simulink model "LQG_CubeSat"  (R2024a)
settings: Solver=VariableStepAuto  StartTime=0.0  StopTime=100  RelTol=1e-3
values from neighbouring files (symbols this model uses):
  I_rw_zz = 0.02 / 523.59    (= 3.81978265437e-05)    [main_CubeSatControl.m]
  I_s = [I_xx 0 0 ... (first row only)    [main_CubeSatControl.m]
  inv_I_s = inv(I_s)    [main_CubeSatControl.m]
  K_p = [K_p_base*axis_ratio 0 0 ... (first row only)    [main_CubeSatControl.m]
  K_pd = [K_pd_base*axis_ratio 0 0 ... (first row only)    [main_CubeSatControl.m]
  tau_motor_loop = 1    [main_CubeSatControl.m]
libraries: vrlib x1, matrix_library x1, aerolibanimutils x1, simulink x1
settings Model: Creator=joshk  LastModifiedBy=joshk
settings RTWCC: GPUComputeCapability=3.5

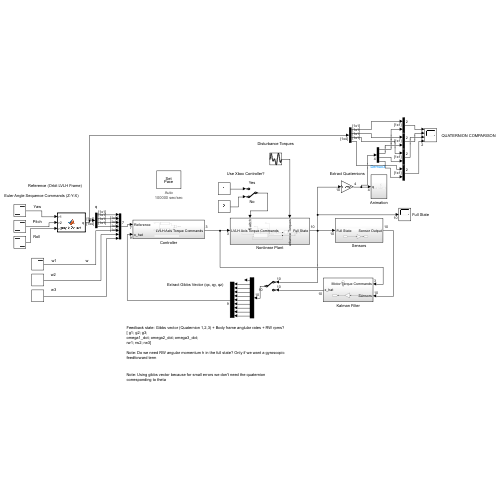
[thumbnail: Simulink's stored preview of the top-level diagram]
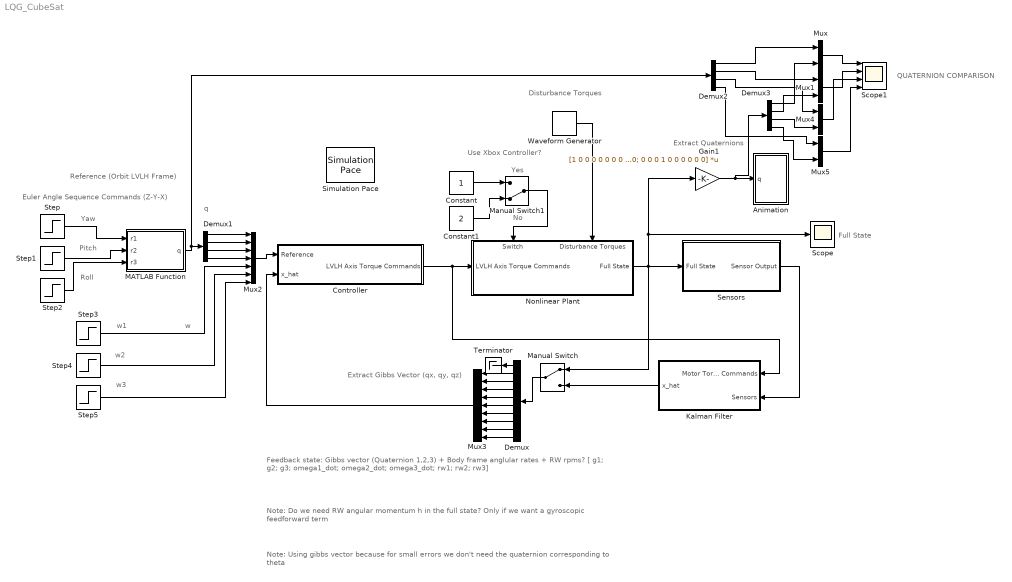
== system LQG_CubeSat ==
  note: QUATERNION COMPARISON
  note: w
  note: q
  note: Disturbance Torques
  note: Note: Using gibbs vector because for small errors we don't need the quaternion corresponding to theta
  note: Full State
  note: Extract Quaternions
  note: Euler Angle Sequence Commands (Z-Y-X)
  note: Note: Do we need RW angular momentum h in the full state? Only if we want a gyroscopic feedforward term
  note: Feedback state: Gibbs vector (Quaternion 1,2,3) + Body frame anglular rates + RW rpms?
      | [ g1; g2; g3;
      | omega1_dot; omega2_dot; omega3_dot;
      | rw1; rw2; rw3]
  note: No
  note: Yes
  note: Use Xbox Controller?
  note: Roll
  note: Pitch
  note: Yaw
  note: Reference (Orbit LVLH Frame)
  note: w2
  note: w3
  note: w1
  note: Extract Gibbs Vector (qx, qy, qz)
  Animation : Subsystem
  Constant : Constant
  Constant1 : Constant  Value=2
  Controller : Subsystem
  Demux : Demux  Outputs=10
  Demux1 : Demux
  Demux2 : Demux
  Demux3 : Demux
  Gain1 : Gain  Gain=[1 0 0 0 0 0 0 0 0 0; 0 1 0 0 0 0 0 0 0 0; 0 0 1 0 0 0 0 0 0 0; 0 0 0 1 0 0 0 0 0 0]  Multiplication=Matrix(K*u) (u vector)
  Kalman Filter : Subsystem
  MATLAB Function : MATLAB Function  TreatAsAtomicUnit=on
  Manual Switch : ManualSwitch
  Manual Switch1 : ManualSwitch  CurrentSetting=0
  Mux{,1,4..5} (4 alike) : Mux  Inputs=2
  Mux2 : Mux  Inputs=7
  Mux3 : Mux  Inputs=9
  Nonlinear Plant : Subsystem
      settings: PortSchema="{\"entries\":[{\"content\":{\"sides\":[{\"content\":{\"connectorIds\":[\"In1\"]},\"type\":\"ConnectorPlacement.EquallySpacedRectSide\",\"uuid\":\"9b91c08c-2a90-4f12-ae99-41b2d0c7dbbf\"},{\"content\":{\"connectorIds\":[\"Out1\"],\"side\":\"RIGHT\"},\"type\":\"ConnectorPlacement.EquallySpacedRectSide\",\"uuid\":\"14ab69da-e910-4abb-8476-8d8dff4f3eb1\"},{\"content\":{\"connectorIds\":[\"In2\",\"In3\"],\"side\":\"TOP\"},\"type\":\"ConnectorPlacement.EquallySpacedRectSide\",\"uuid\":\"c21f965e-6c73-42bc-bf21-433ba90567d6\"}]},\"type\":\"ConnectorPlacement.EquallySpacedConnector\",\"uuid\":\"eb7c3899-db95-4d15-9719-1c6a9ded63d0\"}],\"packageUris\":[\"http://schema.mathworks.com/mf0/Connector/R2020b\"],\"version\":\"1.0\"}"
  Scope : Scope
  Scope1 : Scope  NumInputPorts=4
  Sensors : Subsystem
  Simulation Pace : aerolibanimutils/Simulation Pace  SimulationPace=100000  SleepMode=Auto  OutputPaceError=off  SampleTime=1/50
  Step : Step  Time=2  After=0.1  SampleTime=0
  Step1 : Step  Time=2  After=0.5  SampleTime=0
  Step2 : Step  Time=2  After=-0.3  SampleTime=0
  Step3 : Step  Time=2  After=0  SampleTime=0
  Step4 : Step  Time=2  After=0  SampleTime=0
  Step5 : Step  Time=2  After=0  SampleTime=0
  Terminator : Terminator
  Waveform Generator : simulink/Sources/Waveform Generator  OutMin=[]  OutMax=[]  OutDataTypeStr=double  SelectedSignal=1  BlockNames=MultiportSwitch_e3df3653d217406  SampleTime=0.1
  wires:
  Sensors/1(Sensor Output) -> Kalman Filter/2(Sensors)
  Step1/1 -> MATLAB Function/2(r2)
  Step/1 -> MATLAB Function/1(r1)
  Step2/1 -> MATLAB Function/3(r3)
  Kalman Filter/1(x_hat) -> Manual Switch/2
  Controller/1(LVLH Axis Torque Commands) -> Kalman Filter/1(Motor Torque Commands), Nonlinear Plant/1(LVLH Axis Torque Commands)
  Manual Switch1/1 -> Nonlinear Plant/2(Switch)
  Constant/1 -> Manual Switch1/1
  Constant1/1 -> Manual Switch1/2
  Step5/1 -> Mux2/7
  Step3/1 -> Mux2/5
  Step4/1 -> Mux2/6
  Mux2/1 -> Controller/1(Reference)
  Nonlinear Plant/1(Full State) -> Manual Switch/1, Gain1/1, Scope/1, Sensors/1(Full State)
  Gain1/1 -> Demux3/1, Animation/1(q)
  Manual Switch/1 -> Demux/1
  Demux/2 -> Mux3/1
  Demux/3 -> Mux3/2
  Demux/4 -> Mux3/3
  Demux/5 -> Mux3/4
  Demux/6 -> Mux3/5
  Demux/7 -> Mux3/6
  Demux/8 -> Mux3/7
  Demux/9 -> Mux3/8
  Demux/1 -> Terminator/1
  Mux3/1 -> Controller/2(x_hat)
  Demux/10 -> Mux3/9
  Waveform Generator/1 -> Nonlinear Plant/3(Disturbance Torques)
  MATLAB Function/1(q) -> Demux2/1, Demux1/1
  Demux1/1 -> Mux2/1
  Demux1/2 -> Mux2/2
  Demux1/3 -> Mux2/3
  Demux1/4 -> Mux2/4
  Demux3/1 -> Mux/2
  Demux2/1 -> Mux/1
  Mux/1 -> Scope1/1
  Demux3/2 -> Mux1/2
  Demux2/2 -> Mux1/1
  Mux1/1 -> Scope1/2
  Demux3/3 -> Mux4/2
  Demux2/3 -> Mux4/1
  Mux4/1 -> Scope1/3
  Demux3/4 -> Mux5/2
  Demux2/4 -> Mux5/1
  Mux5/1 -> Scope1/4

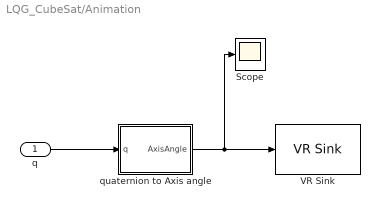
== system LQG_CubeSat/Animation ==
  q : Inport
  Scope : Scope
  VR Sink : vrlib/VR Sink  InstantiateOnLoad=on  SampleTime=0.1  ViewEnable=on  RemoteChange=off  RemoteView=off  FieldsWritten=FBX_LOT__it_fits_together__Transform.rotation.4.1.1.double  WorldFileName=CubeSatEnvironment.x3d  AutoView=off  VideoDimensions=[]  AllowVariableSize=off  FigureProperties="{'Position', 'Name', 'Viewpoint', 'CameraBound', 'CameraDirection', 'CameraPosition', 'CameraUpVector', 'ZoomFactor', 'Antialiasing', 'Headlight', 'Lighting', 'Sound', 'StatusBar', 'Stereo3D', 'Stereo3DCameraOffset', 'Stereo3DHIT', 'ToolBar', 'Textures', 'Transparency', 'Triad', 'Wireframe', 'NavZones', 'NavMode', 'NavSpeed', 'CaptureFileFormat', 'CaptureFileName', 'Record2DCompressMethod', 'Record2DCompressQuality', 'Record2D', 'Record2DFileName', 'Record2DFPS', 'NavPanel'; [1.0000000000000000e+00   1.1560000000000000e+03   1.9200000000000000e+03   3.8800000000000000e+02], '', '_untitled_1', 'on', [0.0000000000000000e+00   0.0000000000000000e+00  -1.0000000000000000e+00], [0.0000000000000000e+00   0.0000000000000000e+00   0.0000000000000000e+00], [0.0000000000000000e+00   1.0000000000000000e+00   0.0000000000000000e+00], [1.0000000000000000e+00], 'on', 'on', 'on', 'on', 'on', 'off', [1.0000000149011612e-01], [0.0000000000000000e+00], 'on', 'on', 'on', 'none', 'off', 'off', 'fly', 'normal', 'tif', '%f_anim_%n.tif', 'auto', [7.5000000000000000e+01], 'off', '%f_anim_%n.avi', 'auto', 'halfbar'}"
  quaternion to Axis angle : MATLAB Function  TreatAsAtomicUnit=on
  wires:
  q/1 -> quaternion to Axis angle/1(q)
  quaternion to Axis angle/1(AxisAngle) -> Scope/1, VR Sink/1

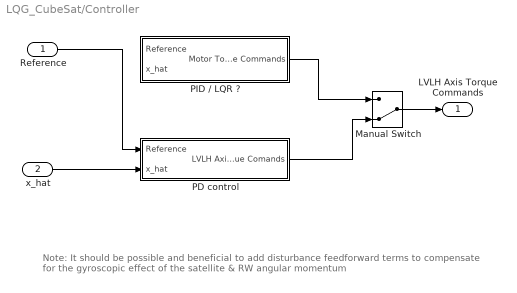
== system LQG_CubeSat/Controller ==
  note: Note: It should be possible and beneficial to add disturbance feedforward terms to compensate for the gyroscopic effect of the satellite & RW angular momentum
  Reference : Inport
  x_hat : Inport  Port=2
  Manual Switch : ManualSwitch  CurrentSetting=0
  PD control : Subsystem
  PID / LQR ? : Subsystem
  LVLH Axis Torque Commands : Outport
  wires:
  Reference/1 -> PD control/1(Reference)
  x_hat/1 -> PD control/2(x_hat)
  PID / LQR ?/1(Motor Torque Commands) -> Manual Switch/1
  Manual Switch/1 -> LVLH Axis Torque Commands/1
  PD control/1(LVLH Axis Torque Comands) -> Manual Switch/2

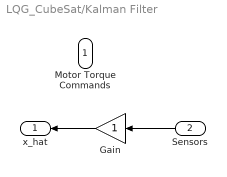
== system LQG_CubeSat/Kalman Filter ==
  Motor Torque Commands : Inport
  Sensors : Inport  Port=2
  Gain : Gain
  x_hat : Outport
  wires:
  Sensors/1 -> Gain/1
  Gain/1 -> x_hat/1

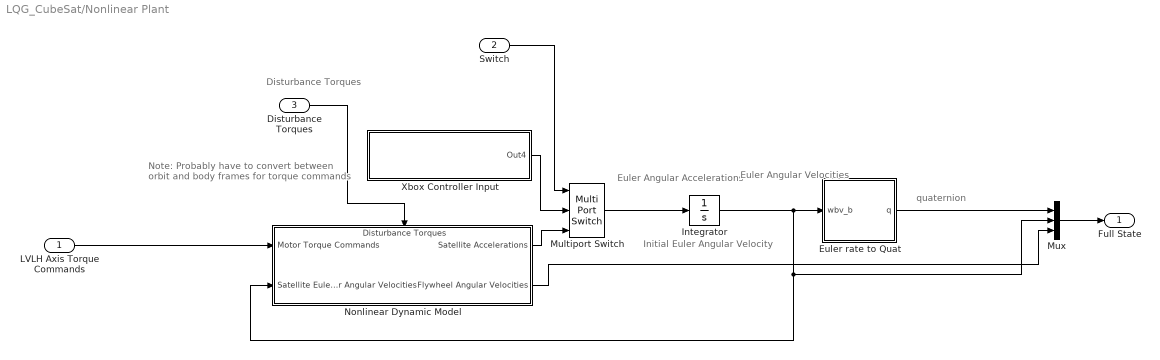
== system LQG_CubeSat/Nonlinear Plant ==
  note: Disturbance Torques
  note: Note: Probably have to convert between orbit and body frames for torque commands
  note: Initial Euler Angular Velocity
  note: Euler Angular Accelerations
  note: quaternion
  note: Euler Angular Velocities
  LVLH Axis Torque Commands : Inport
  Switch : Inport  Port=2
  Disturbance Torques : Inport  Port=3
  Euler rate to Quat : Subsystem
  Integrator : Integrator
  Multiport Switch : MultiPortSwitch  Inputs=2  SaturateOnIntegerOverflow=off  InputSameDT=off
  Mux : Mux  Inputs=3
  Nonlinear Dynamic Model : Subsystem
      settings: PortSchema="{\"entries\":[{\"content\":{\"sides\":[{\"content\":{\"connectorIds\":[\"In1\",\"In2\"]},\"type\":\"ConnectorPlacement.EquallySpacedRectSide\",\"uuid\":\"b133188e-88ab-4812-87e5-a2cae8ba4a28\"},{\"content\":{\"connectorIds\":[\"Out1\",\"Out2\"],\"side\":\"RIGHT\"},\"type\":\"ConnectorPlacement.EquallySpacedRectSide\",\"uuid\":\"aa801b93-c7f4-4f35-9e6f-1c95a6cb7d8e\"},{\"content\":{\"connectorIds\":[\"In3\"],\"side\":\"TOP\"},\"type\":\"ConnectorPlacement.EquallySpacedRectSide\",\"uuid\":\"854fbe33-a555-4bdb-9973-8c05ac9e6acc\"}]},\"type\":\"ConnectorPlacement.EquallySpacedConnector\",\"uuid\":\"327074b1-81b9-4ec3-a55a-9c1b20156f2d\"}],\"packageUris\":[\"http://schema.mathworks.com/mf0/Connector/R2020b\"],\"version\":\"1.0\"}"
  Xbox Controller Input : Subsystem
  Full State : Outport
  wires:
  Xbox Controller Input/1(Out4) -> Multiport Switch/2
  Nonlinear Dynamic Model/1(Satellite Accelerations) -> Multiport Switch/3
  Euler rate to Quat/1(q) -> Mux/1
  Multiport Switch/1 -> Integrator/1
  Integrator/1 -> Nonlinear Dynamic Model/2(Satellite Euler Angular Velocities), Mux/2, Euler rate to Quat/1(wbv_b)
  Mux/1 -> Full State/1
  Nonlinear Dynamic Model/2(Flywheel Angular Velocities) -> Mux/3
  Switch/1 -> Multiport Switch/1
  Disturbance Torques/1 -> Nonlinear Dynamic Model/3(Disturbance Torques)
  LVLH Axis Torque Commands/1 -> Nonlinear Dynamic Model/1(Motor Torque Commands)

== system LQG_CubeSat/Sensors ==
  note: Euler Angle -> Triad Algorithm( Magnetometer + Sun Sensors)
  note: Euler Angular Velocity -> Gyroscope
  note: Flywheel Angular Velocity -> Hall Sensors
  Full State : Inport
  Gain : Gain
  Sensor Output : Outport
  wires:
  Gain/1 -> Sensor Output/1
  Full State/1 -> Gain/1

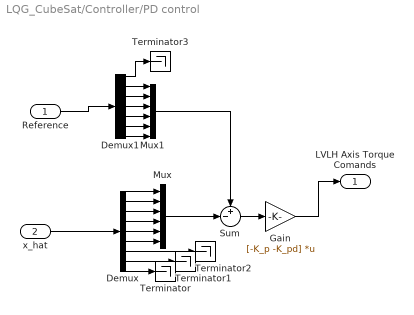
== system LQG_CubeSat/Controller/PD control ==
  Reference : Inport
  x_hat : Inport  Port=2
  Demux : Demux  Outputs=9
  Demux1 : Demux  Outputs=7
  Gain : Gain  Gain=[-K_p -K_pd]  Multiplication=Matrix(K*u) (u vector)
  Mux : Mux  Inputs=6
  Mux1 : Mux  Inputs=6
  Sum : Sum  Inputs=+-|
  Terminator{,1..3} (4 alike) : Terminator
  LVLH Axis Torque Comands : Outport
  wires:
  Demux/7 -> Terminator2/1
  Mux/1 -> Sum/2
  Demux/6 -> Mux/6
  Demux/8 -> Terminator1/1
  Demux/9 -> Terminator/1
  Demux/3 -> Mux/3
  Sum/1 -> Gain/1
  Demux/5 -> Mux/5
  Demux/1 -> Mux/1
  Gain/1 -> LVLH Axis Torque Comands/1
  Demux/2 -> Mux/2
  Demux/4 -> Mux/4
  x_hat/1 -> Demux/1
  Demux1/2 -> Mux1/1
  Demux1/3 -> Mux1/2
  Demux1/4 -> Mux1/3
  Demux1/5 -> Mux1/4
  Demux1/6 -> Mux1/5
  Demux1/7 -> Mux1/6
  Demux1/1 -> Terminator3/1
  Reference/1 -> Demux1/1
  Mux1/1 -> Sum/1

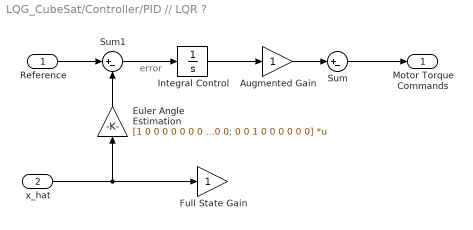
== system LQG_CubeSat/Controller/PID // LQR ? ==
  note: error
  Reference : Inport
  x_hat : Inport  Port=2
  Augmented Gain : Gain
  Euler Angle Estimation : Gain  Gain=[1 0 0 0 0 0 0 0 0; 0 1 0 0 0 0 0 0 0; 0 0 1 0 0 0 0 0 0]  Multiplication=Matrix(K*u) (u vector)
  Full State Gain : Gain
  Integral Control : Integrator
  Sum : Sum  Inputs=|+-
  Sum1 : Sum  Inputs=|+-
  Motor Torque Commands : Outport
  wires:
  Euler Angle Estimation/1 -> Sum1/2
  Augmented Gain/1 -> Sum/1
  x_hat/1 -> Full State Gain/1, Euler Angle Estimation/1
  Sum/1 -> Motor Torque Commands/1
  Integral Control/1 -> Augmented Gain/1
  Reference/1 -> Sum1/1
  Sum1/1 -> Integral Control/1

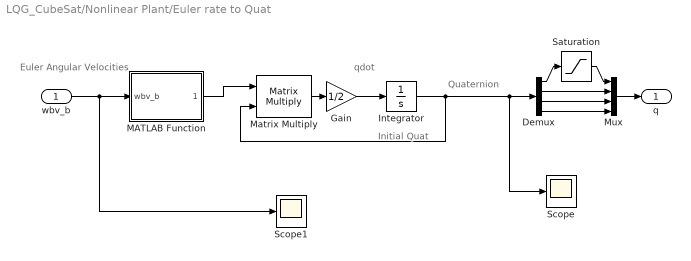
== system LQG_CubeSat/Nonlinear Plant/Euler rate to Quat ==
  note: Initial Quat
  note: Euler Angular Velocities
  note: Quaternion
  note: qdot
  wbv_b : Inport
  Demux : Demux
  Gain : Gain  Gain=1/2
  Integrator : Integrator  InitialCondition=[1 0 0 0]
  MATLAB Function : MATLAB Function  TreatAsAtomicUnit=on
  Matrix Multiply : Product  Multiplication=Matrix(*)
  Mux : Mux
  Saturation : Saturate  UpperLimit=1  LowerLimit=-1
  Scope : Scope
  Scope1 : Scope
  q : Outport
  wires:
  wbv_b/1 -> Scope1/1, MATLAB Function/1(wbv_b)
  MATLAB Function/1(Omega) -> Matrix Multiply/1
  Integrator/1 -> Demux/1, Scope/1, Matrix Multiply/2
  Matrix Multiply/1 -> Gain/1
  Gain/1 -> Integrator/1
  Demux/1 -> Saturation/1
  Saturation/1 -> Mux/1
  Mux/1 -> q/1
  Demux/2 -> Mux/2
  Demux/3 -> Mux/3
  Demux/4 -> Mux/4

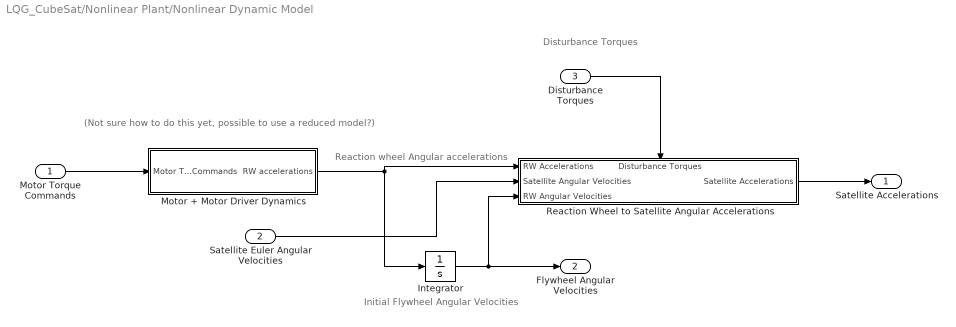
== system LQG_CubeSat/Nonlinear Plant/Nonlinear Dynamic Model ==
  note: Disturbance Torques
  note: (Not sure how to do this yet, possible to use a reduced model?)
  note: Reaction wheel Angular accelerations
  note: Initial Flywheel Angular Velocities
  Motor Torque Commands : Inport
  Satellite Euler Angular Velocities : Inport  Port=2
  Disturbance Torques : Inport  Port=3
  Integrator : Integrator
  Motor + Motor Driver Dynamics : Subsystem
  Reaction Wheel to Satellite Angular Accelerations : Subsystem
      settings: PortSchema="{\"entries\":[{\"content\":{\"sides\":[{\"content\":{\"connectorIds\":[\"In1\",\"In2\",\"In3\"]},\"type\":\"ConnectorPlacement.EquallySpacedRectSide\",\"uuid\":\"f49d1d70-9e85-4e1d-b156-8793e3211305\"},{\"content\":{\"connectorIds\":[\"Out1\"],\"side\":\"RIGHT\"},\"type\":\"ConnectorPlacement.EquallySpacedRectSide\",\"uuid\":\"35de67bb-178b-46d3-aa80-b5d9a68f06e3\"},{\"content\":{\"connectorIds\":[\"In4\"],\"side\":\"TOP\"},\"type\":\"ConnectorPlacement.EquallySpacedRectSide\",\"uuid\":\"55f78edc-5e25-4530-b717-8ca4970259c9\"}]},\"type\":\"ConnectorPlacement.EquallySpacedConnector\",\"uuid\":\"d7035805-976a-40b6-93a5-737fd9e22f36\"}],\"packageUris\":[\"http://schema.mathworks.com/mf0/Connector/R2020b\"],\"version\":\"1.0\"}"
  Satellite Accelerations : Outport
  Flywheel Angular Velocities : Outport  Port=2
  wires:
  Reaction Wheel to Satellite Angular Accelerations/1(Satellite Accelerations) -> Satellite Accelerations/1
  Motor + Motor Driver Dynamics/1(RW accelerations) -> Reaction Wheel to Satellite Angular Accelerations/1(RW Accelerations), Integrator/1
  Motor Torque Commands/1 -> Motor + Motor Driver Dynamics/1(Motor Torque Commands)
  Satellite Euler Angular Velocities/1 -> Reaction Wheel to Satellite Angular Accelerations/2(Satellite Angular Velocities)
  Integrator/1 -> Reaction Wheel to Satellite Angular Accelerations/3(RW Angular Velocities), Flywheel Angular Velocities/1
  Disturbance Torques/1 -> Reaction Wheel to Satellite Angular Accelerations/4(Disturbance Torques)

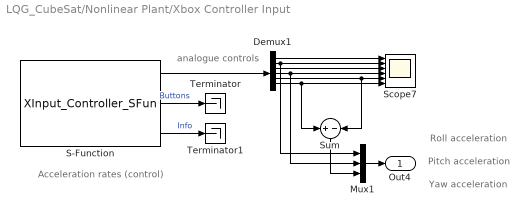
== system LQG_CubeSat/Nonlinear Plant/Xbox Controller Input ==
  note: analogue controls
  note: Roll acceleration
  note: Yaw acceleration
  note: Pitch acceleration
  note: Acceleration rates (control)
  Demux1 : Demux  Outputs=6
  Mux1 : Mux  Inputs=3
  S-Function : S-Function  FunctionName=XInput_Controller_SFun  Parameters=1  SFunctionDeploymentMode=off  EnableBusSupport=off
  Scope7 : Scope  NumInputPorts=6
  Sum : Sum  Inputs=+-
  Terminator : Terminator
  Terminator1 : Terminator
  Out4 : Outport
  wires:
  Demux1/6 -> Scope7/6, Sum/1
  Demux1/2 -> Mux1/1, Scope7/2
  Demux1/5 -> Sum/2, Scope7/5
  Demux1/3 -> Scope7/3
  Demux1/1 -> Scope7/1
  Demux1/4 -> Mux1/2, Scope7/4
  S-Function/1 -> Demux1/1
  Sum/1 -> Mux1/3
  Mux1/1 -> Out4/1
  S-Function/2 -> Terminator/1  "Buttons"
  S-Function/3 -> Terminator1/1  "Info"

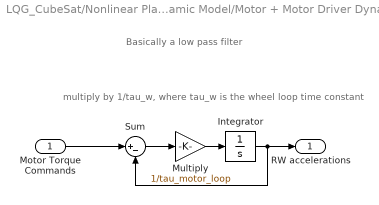
== system LQG_CubeSat/Nonlinear Plant/Nonlinear Dynamic Model/Motor + Motor Driver Dynamics ==
  note: multiply by 1/tau_w, where tau_w is the wheel loop time constant
  note: Basically a low pass filter
  Motor Torque Commands : Inport
  Integrator : Integrator
  Multiply : Gain  Gain=1/tau_motor_loop
  Sum : Sum  Inputs=|+-
  RW accelerations : Outport
  wires:
  Motor Torque Commands/1 -> Sum/1
  Sum/1 -> Multiply/1
  Multiply/1 -> Integrator/1
  Integrator/1 -> Sum/2, RW accelerations/1

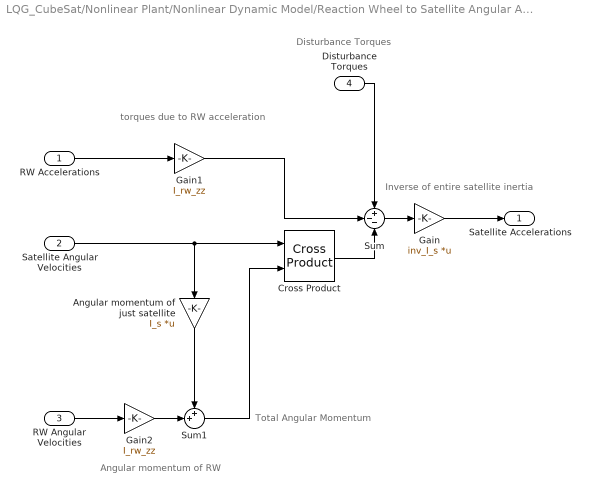
== system LQG_CubeSat/Nonlinear Plant/Nonlinear Dynamic Model/Reaction Wheel to Satellite Angular Accelerations ==
  note: Disturbance Torques
  note: Total Angular Momentum
  note: Angular momentum of RW
  note: torques due to RW acceleration
  note: Inverse of entire satellite inertia
  RW Accelerations : Inport
  Satellite Angular Velocities : Inport  Port=2
  RW Angular Velocities : Inport  Port=3
  Disturbance Torques : Inport  Port=4
  Angular momentum of just satellite : Gain  Gain=I_s  Multiplication=Matrix(K*u) (u vector)
  Cross Product : matrix_library/Cross Product
  Gain : Gain  Gain=inv_I_s  Multiplication=Matrix(K*u) (u vector)
  Gain1 : Gain  Gain=I_rw_zz
  Gain2 : Gain  Gain=I_rw_zz
  Sum : Sum  Inputs=+--
  Sum1 : Sum  Inputs=++|
  Satellite Accelerations : Outport
  wires:
  Gain/1 -> Satellite Accelerations/1
  RW Accelerations/1 -> Gain1/1
  Sum/1 -> Gain/1
  Satellite Angular Velocities/1 -> Angular momentum of just satellite/1, Cross Product/1
  RW Angular Velocities/1 -> Gain2/1
  Gain2/1 -> Sum1/2
  Angular momentum of just satellite/1 -> Sum1/1
  Sum1/1 -> Cross Product/2
  Cross Product/1 -> Sum/3
  Gain1/1 -> Sum/2
  Disturbance Torques/1 -> Sum/1

== matlab function LQG_CubeSat/Animation/quaternion to Axis angle ==
  data: q input; AxisAngle output size=[1 4]
function AxisAngle = fcn(q)

scale = 2*acos(q(1));

x = q(2)/sqrt(1-q(1)^2);
y = q(3)/sqrt(1-q(1)^2);
z = q(4)/sqrt(1-q(1)^2);

AxisAngle = [x,y,z, scale];

== matlab function LQG_CubeSat/Nonlinear Plant/Euler rate to Quat/MATLAB Function ==
  data: wbv_b input; Omega output
function Omega = fcn(wbv_b)
wx = wbv_b(1);
wy = wbv_b(2);
wz = wbv_b(3);


Omega = [...
    0 -wx -wy -wz;
    wx 0 wz -wy;
    wy -wz 0 wx;
    wz wy -wx 0];

== matlab function LQG_CubeSat/MATLAB Function ==
  data: r1 input; q output; r2 input; r3 input
function q = angle2quat( r1, r2, r3)
%  ANGLE2QUAT Convert rotation angles to quaternion.
%   Q = ANGLE2QUAT( R1, R2, R3 ) calculates the quaternion, Q, for given,
%   R1, R2, R3.   R1 is an M array of first rotation angles.  R2 is an M
%   array of second rotation angles.  R3 is an M array of third rotation
%   angles.  Q returns an M-by-4 matrix containing M quaternions. Q has its
%   scalar number as the first column.  Rotation angles are input in radians.    
%
%   Q = ANGLE2QUAT( R1, R2, R3, S ) calculates the quaternion, Q, for a
%   given set of rotation angles, R1, R2, R3, and a specified rotation
%   sequence, S.  
%
%   The default rotation sequence is 'ZYX' where the order of rotation
%   angles for the default rotation are R1 = Z Axis Rotation, R2 = Y Axis
%   Rotation, and R3 = X Axis Rotation. 
%
%   All rotation sequences, S, are supported: 'ZYX', 'ZYZ', 'ZXY', 'ZXZ',
%   'YXZ', 'YXY', 'YZX', 'YZY', 'XYZ', 'XYX', 'XZY', and 'XZX'.
%
%   Examples:
%
%   Determine the quaternion from rotation angles:
%      yaw = 0.7854; 
%      pitch = 0.1; 
%      roll = 0;
%      q = angle2quat( yaw, pitch, roll )
%
%   Determine the quaternions from multiple rotation angles:
%      yaw = [0.7854 0.5]; 
%      pitch = [0.1 0.3]; 
%      roll = [0 0.1];
%      q = angle2quat( pitch, roll, yaw, 'YXZ' )
%
%   See also DCM2QUAT, QUAT2DCM, QUAT2ANGLE.

%   Copyright 2000-2016 The MathWorks, Inc.

narginchk(3,4);

if any(~isreal(r1) || ~isnumeric(r1))
    error(message('aero:angle2quat:isNotReal1'));
end

if any(~isreal(r2) || ~isnumeric(r2))
    error(message('aero:angle2quat:isNotReal2'));
end

if any(~isreal(r3) || ~isnumeric(r3))
    error(message('aero:angle2quat:isNotReal3'));
end

if (length(r1) ~= length(r2)) || (length(r1) ~= length(r3))
    error(message('aero:angle2quat:wrongDimension'));
end

if nargin == 3
    type = 'zyx';
end

angles = [r1(:) r2(:) r3(:)];

cang = cos( angles/2 );
sang = sin( angles/2 );

switch lower( type )
    case 'zyx'
        q = [ cang(:,1).*cang(:,2).*cang(:,3) + sang(:,1).*sang(:,2).*sang(:,3), ...
            cang(:,1).*cang(:,2).*sang(:,3) - sang(:,1).*sang(:,2).*cang(:,3), ...
            cang(:,1).*sang(:,2).*cang(:,3) + sang(:,1).*cang(:,2).*sang(:,3), ...
            sang(:,1).*cang(:,2).*cang(:,3) - cang(:,1).*sang(:,2).*sang(:,3)];
    case 'zyz'
        q = [ cang(:,1).*cang(:,2).*cang(:,3) - sang(:,1).*cang(:,2).*sang(:,3), ...
            cang(:,1).*sang(:,2).*sang(:,3) - sang(:,1).*sang(:,2).*cang(:,3), ...
            cang(:,1).*sang(:,2).*cang(:,3) + sang(:,1).*sang(:,2).*sang(:,3), ...
            sang(:,1).*cang(:,2).*cang(:,3) + cang(:,1).*cang(:,2).*sang(:,3)];
    case 'zxy'
        q = [ cang(:,1).*cang(:,2).*cang(:,3) - sang(:,1).*sang(:,2).*sang(:,3), ...
            cang(:,1).*sang(:,2).*cang(:,3) - sang(:,1).*cang(:,2).*sang(:,3), ...
            cang(:,1).*cang(:,2).*sang(:,3) + sang(:,1).*sang(:,2).*cang(:,3), ...
            cang(:,1).*sang(:,2).*sang(:,3) + sang(:,1).*cang(:,2).*cang(:,3)];
    case 'zxz'
        q = [ cang(:,1).*cang(:,2).*cang(:,3) - sang(:,1).*cang(:,2).*sang(:,3), ...
            cang(:,1).*sang(:,2).*cang(:,3) + sang(:,1).*sang(:,2).*sang(:,3), ...
            sang(:,1).*sang(:,2).*cang(:,3) - cang(:,1).*sang(:,2).*sang(:,3), ...
            cang(:,1).*cang(:,2).*sang(:,3) + sang(:,1).*cang(:,2).*cang(:,3)];
    case 'yxz'
        q = [ cang(:,1).*cang(:,2).*cang(:,3) + sang(:,1).*sang(:,2).*sang(:,3), ...
            cang(:,1).*sang(:,2).*cang(:,3) + sang(:,1).*cang(:,2).*sang(:,3), ...
            sang(:,1).*cang(:,2).*cang(:,3) - cang(:,1).*sang(:,2).*sang(:,3), ...
            cang(:,1).*cang(:,2).*sang(:,3) - sang(:,1).*sang(:,2).*cang(:,3)];
    case 'yxy'
        q = [ cang(:,1).*cang(:,2).*cang(:,3) - sang(:,1).*cang(:,2).*sang(:,3), ...
            cang(:,1).*sang(:,2).*cang(:,3) + sang(:,1).*sang(:,2).*sang(:,3), ...
            sang(:,1).*cang(:,2).*cang(:,3) + cang(:,1).*cang(:,2).*sang(:,3), ...
            cang(:,1).*sang(:,2).*sang(:,3) - sang(:,1).*sang(:,2).*cang(:,3)];
    case 'yzx'
        q = [ cang(:,1).*cang(:,2).*cang(:,3) - sang(:,1).*sang(:,2).*sang(:,3), ...
            cang(:,1).*cang(:,2).*sang(:,3) + sang(:,1).*sang(:,2).*cang(:,3), ...
            cang(:,1).*sang(:,2).*sang(:,3) + sang(:,1).*cang(:,2).*cang(:,3), ...
            cang(:,1).*sang(:,2).*cang(:,3) - sang(:,1).*cang(:,2).*sang(:,3)];
    case 'yzy'
        q = [ cang(:,1).*cang(:,2).*cang(:,3) - sang(:,1).*cang(:,2).*sang(:,3), ...
            sang(:,1).*sang(:,2).*cang(:,3) - cang(:,1).*sang(:,2).*sang(:,3), ...
            cang(:,1).*cang(:,2).*sang(:,3) + sang(:,1).*cang(:,2).*cang(:,3), ...
            cang(:,1).*sang(:,2).*cang(:,3) + sang(:,1).*sang(:,2).*sang(:,3)];
    case 'xyz'
        q = [ cang(:,1).*cang(:,2).*cang(:,3) - sang(:,1).*sang(:,2).*sang(:,3), ...
            cang(:,1).*sang(:,2).*sang(:,3) + sang(:,1).*cang(:,2).*cang(:,3), ...
            cang(:,1).*sang(:,2).*cang(:,3) - sang(:,1).*cang(:,2).*sang(:,3), ...
            cang(:,1).*cang(:,2).*sang(:,3) + sang(:,1).*sang(:,2).*cang(:,3)];
    case 'xyx'
        q = [ cang(:,1).*cang(:,2).*cang(:,3) - sang(:,1).*cang(:,2).*sang(:,3), ...
            cang(:,1).*cang(:,2).*sang(:,3) + sang(:,1).*cang(:,2).*cang(:,3), ...
            cang(:,1).*sang(:,2).*cang(:,3) + sang(:,1).*sang(:,2).*sang(:,3), ...
            sang(:,1).*sang(:,2).*cang(:,3) - cang(:,1).*sang(:,2).*sang(:,3)];
    case 'xzy'
        q = [ cang(:,1).*cang(:,2).*cang(:,3) + sang(:,1).*sang(:,2).*sang(:,3), ...
            sang(:,1).*cang(:,2).*cang(:,3) - cang(:,1).*sang(:,2).*sang(:,3), ...
            cang(:,1).*cang(:,2).*sang(:,3) - sang(:,1).*sang(:,2).*cang(:,3), ...
            cang(:,1).*sang(:,2).*cang(:,3) + sang(:,1).*cang(:,2).*sang(:,3)];
    case 'xzx'
        q = [ cang(:,1).*cang(:,2).*cang(:,3) - sang(:,1).*cang(:,2).*sang(:,3), ...
            cang(:,1).*cang(:,2).*sang(:,3) + sang(:,1).*cang(:,2).*cang(:,3), ...
            cang(:,1).*sang(:,2).*sang(:,3) - sang(:,1).*sang(:,2).*cang(:,3), ...
            cang(:,1).*sang(:,2).*cang(:,3) + sang(:,1).*sang(:,2).*sang(:,3)];
    otherwise
        error(message('aero:angle2quat:unknownRotation', type));
end
